simulink model "P_controller"  (R2019b)
settings: Solver=VariableStepAuto  StartTime=0.0  StopTime=10.0  RelTol=1e-3
values from neighbouring files (symbols this model uses):
  P1 = COEF_P1*K_kr    [code6.m]
settings Model: Creator=Szymon  LastModifiedBy=Szymon

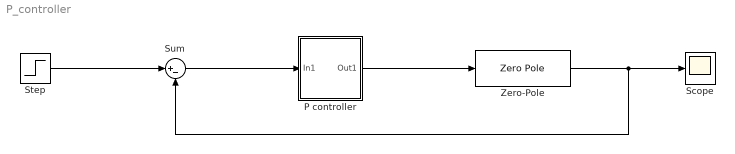
== system P_controller ==
  P controller : Subsystem  mask{P=P1}
  Scope : Scope
  Step : Step  SampleTime=0
  Sum : Sum  Inputs=|+-
  Zero-Pole : ZeroPole  Zeros=[]  Poles=[-1 -1 -1]
  wires:
  Sum/1 -> P controller/1(In1)
  P controller/1(Out1) -> Zero-Pole/1
  Step/1 -> Sum/1
  Zero-Pole/1 -> Sum/2, Scope/1

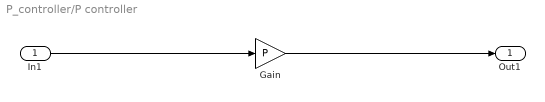
== system P_controller/P controller ==
  In1 : Inport
  Gain : Gain  Gain=P
  Out1 : Outport
  wires:
  Gain/1 -> Out1/1
  In1/1 -> Gain/1
